simulink model "MathOperator_Demo"  (R2017b)
settings: Solver=VariableStepAuto  StartTime=0.0  StopTime=10.0  RelTol=1e-3
settings Model: Creator=javed  LastModifiedBy=javed

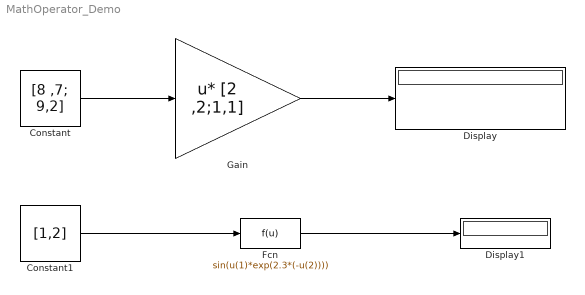
== system MathOperator_Demo ==
  Constant : Constant  Value=[8 ,7; 9,2]
  Constant1 : Constant  Value=[1,2]
  Display : Display
  Display1 : Display
  Fcn : Fcn  Expr=sin(u(1)*exp(2.3*(-u(2))))
  Gain : Gain  Gain=[2 ,2;1,1]  Multiplication=Matrix(u*K)
  wires:
  Constant/1 -> Gain/1
  Gain/1 -> Display/1
  Constant1/1 -> Fcn/1
  Fcn/1 -> Display1/1
